simulink model "Control_v2"  (R2019b)
settings: Solver=FixedStepAuto  StartTime=0.0  StopTime=10  FixedStep=str2num(Step_size)  RelTol=1e-3
model workspace: external: MATLAB File H:\4-project\matlab\github\Sim-v2\bicopter_sim\Bicopter_DataFile14.m (data not in the file)
values from neighbouring files (symbols this model uses):
  b = [5,1,5,4]    [init_ADRC_val.m]    (also in init_Non_Linear_ADRC_val.m = 0.5*[1,    1, 6,  6]')
  b_sep = gains(5:8)    [get_ADRC_parameters.m]    (also in get_adrc_sep.m = [  2   7    6   7]; get_adrc_sep_kalman.m = [  2   2    6   7])
  C = [eye(4),zeros(4,8)]    [init_ADRC_val.m]
  C_air = 0.0025    [Sim_Script.m]
  d_f_phi = 100    [Sim_Script.m]
  d_f_psi = 25    [Sim_Script.m]
  d_f_theta = 10    [Sim_Script.m]
  d_f_z = 100    [Sim_Script.m]
  eps_sep = 0.7*[1 1 1 1]    [get_ADRC_parameters.m]    (also in get_adrc_sep.m = [0.7 0.3 0.3 0.35]; get_adrc_sep_kalman.m = [0.7 0.7 0.3 0.35])
  epsi = 1.5    [init_Non_Linear_ADRC_val.m]
  euler_source = 1    [Sim_Script.m]
  freq_cut_angvel_phi = 75    [Sim_Script.m]
  freq_cut_angvel_psi = 75    [Sim_Script.m]
  freq_cut_angvel_theta = 50    [Sim_Script.m]
  g = 9.81    [Sim_Script.m]
  K = place(A1,B1,w00(1:8))    [init_ADRC_val.m]
  L = place(A',C',8*w00)'    [init_ADRC_val.m]
  method = STSC_controller    (= 2)    [Sim_Script.m]
  method_angle_plane_sw = plane_sw    (= 2)    [Sim_Script.m]
  mult_obs = 10    [init_Non_Linear_ADRC_val.m]
  Noise_gain = 1    [Sim_Script.m]
  PID_VAL_SEP = init_pid_val_sep()    [Sim_Script.m]
  polarity = [-1;1;1;1]    [Sim_Script.m]
  r = [10,5,10,10]    [init_Non_Linear_ADRC_val.m]
  S_phi = 0.001    [Sim_Script.m]
  S_psi = S_phi    (= 0.001)    [Sim_Script.m]
  S_theta = S_phi    (= 0.001)    [Sim_Script.m]
  State_step = [Z_step;Phi_step;Theta_step;Psi_step]    [req_response.m]
  Step_size = step_size    [Sim_Script.m]
  STSC_VAL = init_STSC_val()    [Sim_Script.m]
  time_delay = 1e-6    (= 1e-06)    [Sim_Script.m]
  V_phi = 0.01    [Sim_Script.m]
  V_psi = 0.01    [Sim_Script.m]
  V_theta = 0.01    [Sim_Script.m]
  wc_sep = gains(1:4)    [get_ADRC_parameters.m]    (also in get_adrc_sep.m = [ 5.54   9   6    3]; get_adrc_sep_kalman.m = [ 5.54   9   6    3])
  wo_sep = ga*wc_sep    [get_ADRC_parameters.m]    (also in get_adrc_sep.m; get_adrc_sep_kalman.m)
undefined symbols (not defined in the file or in its folder): Continuous, magnitude, NLADRC_VAL, sigbuilder_block, smiData, Time, X, Y, Z
libraries: sm_lib x141, nesl_utility x20, simulink x19, fuzblock x3, sharedtransform x1, ctrlSharedLib x1
(part 6 of 7)

== system Control_v2/System/Controller/fuzzy logic/inner_loop1 ==
  note: Scope_P
  err : Inport
  y_dot : Inport  Port=2
  Derivative : Derivative
  Gain : Gain  Gain=PID_VAL_SEP(parm_id,3)
  Gain1 : Gain  Gain=PID_VAL_SEP(parm_id,3)
  Gain2 : Gain  Gain=PID_VAL_SEP(parm_id,2)
  I : simulink/Continuous/PID Controller  Controller=PID  Form=Parallel  TimeDomain=Continuous-time  SampleTime=-1  IntegratorMethod=Forward Euler  FilterMethod=Forward Euler  ControllerParametersSource=internal  P=0  I=PID_VAL_SEP(parm_id,2)  D=0  UseFilter=on  N=0  TunerSelectOption=Transfer Function Based (PID Tuner App)  InitialConditionSource=internal  InitialConditionForIntegrator=0  InitialConditionForFilter=0  DifferentiatorICPrevScaledInput=0  ExternalReset=none  TrackingMode=off  Kt=1  LimitOutput=off  UpperSaturationLimit=inf  LowerSaturationLimit=-inf  LinearizeAsGain=on  AntiWindupMode=none  Kb=1  POutMin=[]  POutMax=[]  IOutMin=[]  IOutMax=[]  DOutMin=[]  DOutMax=[]  NOutMin=[]  NOutMax=[]  SumOutMin=[]  SumOutMax=[]  SaturationOutMin=[]  SaturationOutMax=[]  PParamMin=[]  PParamMax=[]  IParamMin=[]  IParamMax=[]  DParamMin=[]  DParamMax=[]  NParamMin=[]  NParamMax=[]  KbParamMin=[]  KbParamMax=[]  KtParamMin=[]  KtParamMax=[]  KbOutMin=[]  KbOutMax=[]  KtOutMin=[]  KtOutMax=[]  IntegratorOutMin=[]  IntegratorOutMax=[]  FilterOutMin=[]  FilterOutMax=[]  SumI1OutMin=[]  SumI1OutMax=[]  SumI2OutMin=[]  SumI2OutMax=[]  SumI3OutMin=[]  SumI3OutMax=[]  SumI4OutMin=[]  SumI4OutMax=[]  SumDOutMin=[]  SumDOutMax=[]  DifferentiatorOutMin=[]  DifferentiatorOutMax=[]  FilterDiffOutCoefMin=[]  FilterDiffOutCoefMax=[]  ReciprocalOutMin=[]  ReciprocalOutMax=[]  SumDenOutMin=[]  SumDenOutMax=[]  SumNumOutMin=[]  SumNumOutMax=[]  DivideOutMin=[]  DivideOutMax=[]  IntegratorContinuousStateAttributes=''  IntegratorStateMustResolveToSignalObject=off  IntegratorRTWStateStorageClass=Auto  FilterContinuousStateAttributes=''  FilterStateMustResolveToSignalObject=off  FilterRTWStateStorageClass=Auto  ParallelPVariant=InternalParameters  IdealPVariant=Disabled  IVariant=InternalParameters  DVariant=InternalParameters  IntegratorVariant=Continuous  SatVariant=Disabled  AWVariant=Passthrough  PCopyVariant=Disabled  TRVariant=Disabled  FdbkBlocksVariant=Forward  IdealPFdbkVariant=Disabled  SatFdbkVariant=Disabled  DerivativeFilterVariant=ContFilter  NVariant=InternalParameters  NCopyVariant=Disabled  FilterICVariant=InternalICsFilter  IntegratorICVariant=InternalICs  ExternalResetVariant=Disabled  TRSumVariant=Passthrough  SumFdbkVariant=Disabled  SumVariant=Sum_PID
  Integrator Limited : Integrator  LimitOutput=on  UpperSaturationLimit=5  LowerSaturationLimit=-5
  P : simulink/Continuous/PID Controller  Controller=PID  Form=Parallel  TimeDomain=Continuous-time  SampleTime=-1  IntegratorMethod=Forward Euler  FilterMethod=Forward Euler  ControllerParametersSource=internal  P=PID_VAL_SEP(parm_id,1)  I=0  D=0  UseFilter=on  N=0  TunerSelectOption=Transfer Function Based (PID Tuner App)  InitialConditionSource=internal  InitialConditionForIntegrator=0  InitialConditionForFilter=0  DifferentiatorICPrevScaledInput=0  ExternalReset=none  TrackingMode=off  Kt=1  LimitOutput=off  UpperSaturationLimit=inf  LowerSaturationLimit=-inf  LinearizeAsGain=on  AntiWindupMode=none  Kb=1  POutMin=[]  POutMax=[]  IOutMin=[]  IOutMax=[]  DOutMin=[]  DOutMax=[]  NOutMin=[]  NOutMax=[]  SumOutMin=[]  SumOutMax=[]  SaturationOutMin=[]  SaturationOutMax=[]  PParamMin=[]  PParamMax=[]  IParamMin=[]  IParamMax=[]  DParamMin=[]  DParamMax=[]  NParamMin=[]  NParamMax=[]  KbParamMin=[]  KbParamMax=[]  KtParamMin=[]  KtParamMax=[]  KbOutMin=[]  KbOutMax=[]  KtOutMin=[]  KtOutMax=[]  IntegratorOutMin=[]  IntegratorOutMax=[]  FilterOutMin=[]  FilterOutMax=[]  SumI1OutMin=[]  SumI1OutMax=[]  SumI2OutMin=[]  SumI2OutMax=[]  SumI3OutMin=[]  SumI3OutMax=[]  SumI4OutMin=[]  SumI4OutMax=[]  SumDOutMin=[]  SumDOutMax=[]  DifferentiatorOutMin=[]  DifferentiatorOutMax=[]  FilterDiffOutCoefMin=[]  FilterDiffOutCoefMax=[]  ReciprocalOutMin=[]  ReciprocalOutMax=[]  SumDenOutMin=[]  SumDenOutMax=[]  SumNumOutMin=[]  SumNumOutMax=[]  DivideOutMin=[]  DivideOutMax=[]  IntegratorContinuousStateAttributes=''  IntegratorStateMustResolveToSignalObject=off  IntegratorRTWStateStorageClass=Auto  FilterContinuousStateAttributes=''  FilterStateMustResolveToSignalObject=off  FilterRTWStateStorageClass=Auto  ParallelPVariant=InternalParameters  IdealPVariant=Disabled  IVariant=InternalParameters  DVariant=InternalParameters  IntegratorVariant=Continuous  SatVariant=Disabled  AWVariant=Passthrough  PCopyVariant=Disabled  TRVariant=Disabled  FdbkBlocksVariant=Forward  IdealPFdbkVariant=Disabled  SatFdbkVariant=Disabled  DerivativeFilterVariant=ContFilter  NVariant=InternalParameters  NCopyVariant=Disabled  FilterICVariant=InternalICsFilter  IntegratorICVariant=InternalICs  ExternalResetVariant=Disabled  TRSumVariant=Passthrough  SumFdbkVariant=Disabled  SumVariant=Sum_PID
  Scope : Scope  NumInputPorts=2
  Scope1 : Scope  NumInputPorts=2
  Scope_D : Scope  NumInputPorts=2
  Scope_D1 : Scope  NumInputPorts=2
  Scope_I : Scope  NumInputPorts=2
  Sum : Sum  Inputs=|+++-
  Transfer Fcn : TransferFcn  Numerator=[2*pi*f]  Denominator=[1 2*pi*f]
  Transfer Fcn1 : TransferFcn  Numerator=[2*pi*f]  Denominator=[1 2*pi*f]
  phiCmd : Scope  NumInputPorts=2
  cmd : Outport
  wires:
  Sum/1 -> phiCmd/2, cmd/1  "after"
  y_dot/1 -> Gain/1, Scope_D/1
  err/1 -> Gain2/1, Gain1/1, I/1, Scope_I/2, P/1, Scope/1, phiCmd/1  "err"
  P/1 -> Sum/1, Scope/2
  I/1 -> Scope1/2, Scope_I/1
  Gain1/1 -> Derivative/1  "before"
  Derivative/1 -> Transfer Fcn/1
  Gain/1 -> Sum/4, Transfer Fcn1/1  "before"
  Gain2/1 -> Integrator Limited/1
  Integrator Limited/1 -> Scope1/1, Sum/3

== system Control_v2/System/Controller/fuzzy logic/inner_loop2 ==
  note: Scope_P
  err : Inport
  y_dot : Inport  Port=2
  Derivative : Derivative
  Gain : Gain  Gain=PID_VAL_SEP(parm_id,3)
  Gain1 : Gain  Gain=PID_VAL_SEP(parm_id,3)
  I : simulink/Continuous/PID Controller  Controller=PID  Form=Parallel  TimeDomain=Continuous-time  SampleTime=-1  IntegratorMethod=Forward Euler  FilterMethod=Forward Euler  ControllerParametersSource=internal  P=0  I=PID_VAL_SEP(parm_id,2)  D=0  UseFilter=on  N=0  TunerSelectOption=Transfer Function Based (PID Tuner App)  InitialConditionSource=internal  InitialConditionForIntegrator=0  InitialConditionForFilter=0  DifferentiatorICPrevScaledInput=0  ExternalReset=none  TrackingMode=off  Kt=1  LimitOutput=off  UpperSaturationLimit=inf  LowerSaturationLimit=-inf  LinearizeAsGain=on  AntiWindupMode=none  Kb=1  POutMin=[]  POutMax=[]  IOutMin=[]  IOutMax=[]  DOutMin=[]  DOutMax=[]  NOutMin=[]  NOutMax=[]  SumOutMin=[]  SumOutMax=[]  SaturationOutMin=[]  SaturationOutMax=[]  PParamMin=[]  PParamMax=[]  IParamMin=[]  IParamMax=[]  DParamMin=[]  DParamMax=[]  NParamMin=[]  NParamMax=[]  KbParamMin=[]  KbParamMax=[]  KtParamMin=[]  KtParamMax=[]  KbOutMin=[]  KbOutMax=[]  KtOutMin=[]  KtOutMax=[]  IntegratorOutMin=[]  IntegratorOutMax=[]  FilterOutMin=[]  FilterOutMax=[]  SumI1OutMin=[]  SumI1OutMax=[]  SumI2OutMin=[]  SumI2OutMax=[]  SumI3OutMin=[]  SumI3OutMax=[]  SumI4OutMin=[]  SumI4OutMax=[]  SumDOutMin=[]  SumDOutMax=[]  DifferentiatorOutMin=[]  DifferentiatorOutMax=[]  FilterDiffOutCoefMin=[]  FilterDiffOutCoefMax=[]  ReciprocalOutMin=[]  ReciprocalOutMax=[]  SumDenOutMin=[]  SumDenOutMax=[]  SumNumOutMin=[]  SumNumOutMax=[]  DivideOutMin=[]  DivideOutMax=[]  IntegratorContinuousStateAttributes=''  IntegratorStateMustResolveToSignalObject=off  IntegratorRTWStateStorageClass=Auto  FilterContinuousStateAttributes=''  FilterStateMustResolveToSignalObject=off  FilterRTWStateStorageClass=Auto  ParallelPVariant=InternalParameters  IdealPVariant=Disabled  IVariant=InternalParameters  DVariant=InternalParameters  IntegratorVariant=Continuous  SatVariant=Disabled  AWVariant=Passthrough  PCopyVariant=Disabled  TRVariant=Disabled  FdbkBlocksVariant=Forward  IdealPFdbkVariant=Disabled  SatFdbkVariant=Disabled  DerivativeFilterVariant=ContFilter  NVariant=InternalParameters  NCopyVariant=Disabled  FilterICVariant=InternalICsFilter  IntegratorICVariant=InternalICs  ExternalResetVariant=Disabled  TRSumVariant=Passthrough  SumFdbkVariant=Disabled  SumVariant=Sum_PID
  P : simulink/Continuous/PID Controller  Controller=PID  Form=Parallel  TimeDomain=Continuous-time  SampleTime=-1  IntegratorMethod=Forward Euler  FilterMethod=Forward Euler  ControllerParametersSource=internal  P=PID_VAL_SEP(parm_id,1)  I=0  D=0  UseFilter=on  N=0  TunerSelectOption=Transfer Function Based (PID Tuner App)  InitialConditionSource=internal  InitialConditionForIntegrator=0  InitialConditionForFilter=0  DifferentiatorICPrevScaledInput=0  ExternalReset=none  TrackingMode=off  Kt=1  LimitOutput=off  UpperSaturationLimit=inf  LowerSaturationLimit=-inf  LinearizeAsGain=on  AntiWindupMode=none  Kb=1  POutMin=[]  POutMax=[]  IOutMin=[]  IOutMax=[]  DOutMin=[]  DOutMax=[]  NOutMin=[]  NOutMax=[]  SumOutMin=[]  SumOutMax=[]  SaturationOutMin=[]  SaturationOutMax=[]  PParamMin=[]  PParamMax=[]  IParamMin=[]  IParamMax=[]  DParamMin=[]  DParamMax=[]  NParamMin=[]  NParamMax=[]  KbParamMin=[]  KbParamMax=[]  KtParamMin=[]  KtParamMax=[]  KbOutMin=[]  KbOutMax=[]  KtOutMin=[]  KtOutMax=[]  IntegratorOutMin=[]  IntegratorOutMax=[]  FilterOutMin=[]  FilterOutMax=[]  SumI1OutMin=[]  SumI1OutMax=[]  SumI2OutMin=[]  SumI2OutMax=[]  SumI3OutMin=[]  SumI3OutMax=[]  SumI4OutMin=[]  SumI4OutMax=[]  SumDOutMin=[]  SumDOutMax=[]  DifferentiatorOutMin=[]  DifferentiatorOutMax=[]  FilterDiffOutCoefMin=[]  FilterDiffOutCoefMax=[]  ReciprocalOutMin=[]  ReciprocalOutMax=[]  SumDenOutMin=[]  SumDenOutMax=[]  SumNumOutMin=[]  SumNumOutMax=[]  DivideOutMin=[]  DivideOutMax=[]  IntegratorContinuousStateAttributes=''  IntegratorStateMustResolveToSignalObject=off  IntegratorRTWStateStorageClass=Auto  FilterContinuousStateAttributes=''  FilterStateMustResolveToSignalObject=off  FilterRTWStateStorageClass=Auto  ParallelPVariant=InternalParameters  IdealPVariant=Disabled  IVariant=InternalParameters  DVariant=InternalParameters  IntegratorVariant=Continuous  SatVariant=Disabled  AWVariant=Passthrough  PCopyVariant=Disabled  TRVariant=Disabled  FdbkBlocksVariant=Forward  IdealPFdbkVariant=Disabled  SatFdbkVariant=Disabled  DerivativeFilterVariant=ContFilter  NVariant=InternalParameters  NCopyVariant=Disabled  FilterICVariant=InternalICsFilter  IntegratorICVariant=InternalICs  ExternalResetVariant=Disabled  TRSumVariant=Passthrough  SumFdbkVariant=Disabled  SumVariant=Sum_PID
  Scope : Scope  NumInputPorts=2
  Scope_D : Scope  NumInputPorts=2
  Scope_D1 : Scope  NumInputPorts=2
  Scope_I : Scope  NumInputPorts=2
  Sum : Sum  Inputs=|+++-
  Transfer Fcn : TransferFcn  Numerator=[2*pi*f]  Denominator=[1 2*pi*f]
  Transfer Fcn1 : TransferFcn  Numerator=[2*pi*f]  Denominator=[1 2*pi*f]
  phiCmd : Scope  NumInputPorts=2
  cmd : Outport
  wires:
  Gain/1 -> Transfer Fcn1/1  "before"
  I/1 -> Scope_I/1, Sum/2
  P/1 -> Scope/2, Sum/1
  err/1 -> phiCmd/1, Gain1/1, Scope/1, P/1, Scope_I/2, I/1  "err"
  y_dot/1 -> Gain/1
  Sum/1 -> cmd/1, phiCmd/2  "after"
  Derivative/1 -> Scope_D/2, Transfer Fcn/1
  Gain1/1 -> Derivative/1  "before"
  Transfer Fcn/1 -> Scope_D/1  "after"
  Transfer Fcn1/1 -> Scope_D1/2, Sum/4  "after"

== system Control_v2/System/Controller/fuzzy logic/inner_loop4 ==
  note: Scope_P
  err : Inport
  y_dot : Inport  Port=2
  Derivative : Derivative
  Gain : Gain  Gain=PID_VAL_SEP(parm_id,3)
  Gain1 : Gain  Gain=PID_VAL_SEP(parm_id,3)
  I : simulink/Continuous/PID Controller  Controller=PID  Form=Parallel  TimeDomain=Continuous-time  SampleTime=-1  IntegratorMethod=Forward Euler  FilterMethod=Forward Euler  ControllerParametersSource=internal  P=0  I=PID_VAL_SEP(parm_id,2)  D=0  UseFilter=on  N=0  TunerSelectOption=Transfer Function Based (PID Tuner App)  InitialConditionSource=internal  InitialConditionForIntegrator=0  InitialConditionForFilter=0  DifferentiatorICPrevScaledInput=0  ExternalReset=none  TrackingMode=off  Kt=1  LimitOutput=off  UpperSaturationLimit=inf  LowerSaturationLimit=-inf  LinearizeAsGain=on  AntiWindupMode=none  Kb=1  POutMin=[]  POutMax=[]  IOutMin=[]  IOutMax=[]  DOutMin=[]  DOutMax=[]  NOutMin=[]  NOutMax=[]  SumOutMin=[]  SumOutMax=[]  SaturationOutMin=[]  SaturationOutMax=[]  PParamMin=[]  PParamMax=[]  IParamMin=[]  IParamMax=[]  DParamMin=[]  DParamMax=[]  NParamMin=[]  NParamMax=[]  KbParamMin=[]  KbParamMax=[]  KtParamMin=[]  KtParamMax=[]  KbOutMin=[]  KbOutMax=[]  KtOutMin=[]  KtOutMax=[]  IntegratorOutMin=[]  IntegratorOutMax=[]  FilterOutMin=[]  FilterOutMax=[]  SumI1OutMin=[]  SumI1OutMax=[]  SumI2OutMin=[]  SumI2OutMax=[]  SumI3OutMin=[]  SumI3OutMax=[]  SumI4OutMin=[]  SumI4OutMax=[]  SumDOutMin=[]  SumDOutMax=[]  DifferentiatorOutMin=[]  DifferentiatorOutMax=[]  FilterDiffOutCoefMin=[]  FilterDiffOutCoefMax=[]  ReciprocalOutMin=[]  ReciprocalOutMax=[]  SumDenOutMin=[]  SumDenOutMax=[]  SumNumOutMin=[]  SumNumOutMax=[]  DivideOutMin=[]  DivideOutMax=[]  IntegratorContinuousStateAttributes=''  IntegratorStateMustResolveToSignalObject=off  IntegratorRTWStateStorageClass=Auto  FilterContinuousStateAttributes=''  FilterStateMustResolveToSignalObject=off  FilterRTWStateStorageClass=Auto  ParallelPVariant=InternalParameters  IdealPVariant=Disabled  IVariant=InternalParameters  DVariant=InternalParameters  IntegratorVariant=Continuous  SatVariant=Disabled  AWVariant=Passthrough  PCopyVariant=Disabled  TRVariant=Disabled  FdbkBlocksVariant=Forward  IdealPFdbkVariant=Disabled  SatFdbkVariant=Disabled  DerivativeFilterVariant=ContFilter  NVariant=InternalParameters  NCopyVariant=Disabled  FilterICVariant=InternalICsFilter  IntegratorICVariant=InternalICs  ExternalResetVariant=Disabled  TRSumVariant=Passthrough  SumFdbkVariant=Disabled  SumVariant=Sum_PID
  P : simulink/Continuous/PID Controller  Controller=PID  Form=Parallel  TimeDomain=Continuous-time  SampleTime=-1  IntegratorMethod=Forward Euler  FilterMethod=Forward Euler  ControllerParametersSource=internal  P=PID_VAL_SEP(parm_id,1)  I=0  D=0  UseFilter=on  N=0  TunerSelectOption=Transfer Function Based (PID Tuner App)  InitialConditionSource=internal  InitialConditionForIntegrator=0  InitialConditionForFilter=0  DifferentiatorICPrevScaledInput=0  ExternalReset=none  TrackingMode=off  Kt=1  LimitOutput=off  UpperSaturationLimit=inf  LowerSaturationLimit=-inf  LinearizeAsGain=on  AntiWindupMode=none  Kb=1  POutMin=[]  POutMax=[]  IOutMin=[]  IOutMax=[]  DOutMin=[]  DOutMax=[]  NOutMin=[]  NOutMax=[]  SumOutMin=[]  SumOutMax=[]  SaturationOutMin=[]  SaturationOutMax=[]  PParamMin=[]  PParamMax=[]  IParamMin=[]  IParamMax=[]  DParamMin=[]  DParamMax=[]  NParamMin=[]  NParamMax=[]  KbParamMin=[]  KbParamMax=[]  KtParamMin=[]  KtParamMax=[]  KbOutMin=[]  KbOutMax=[]  KtOutMin=[]  KtOutMax=[]  IntegratorOutMin=[]  IntegratorOutMax=[]  FilterOutMin=[]  FilterOutMax=[]  SumI1OutMin=[]  SumI1OutMax=[]  SumI2OutMin=[]  SumI2OutMax=[]  SumI3OutMin=[]  SumI3OutMax=[]  SumI4OutMin=[]  SumI4OutMax=[]  SumDOutMin=[]  SumDOutMax=[]  DifferentiatorOutMin=[]  DifferentiatorOutMax=[]  FilterDiffOutCoefMin=[]  FilterDiffOutCoefMax=[]  ReciprocalOutMin=[]  ReciprocalOutMax=[]  SumDenOutMin=[]  SumDenOutMax=[]  SumNumOutMin=[]  SumNumOutMax=[]  DivideOutMin=[]  DivideOutMax=[]  IntegratorContinuousStateAttributes=''  IntegratorStateMustResolveToSignalObject=off  IntegratorRTWStateStorageClass=Auto  FilterContinuousStateAttributes=''  FilterStateMustResolveToSignalObject=off  FilterRTWStateStorageClass=Auto  ParallelPVariant=InternalParameters  IdealPVariant=Disabled  IVariant=InternalParameters  DVariant=InternalParameters  IntegratorVariant=Continuous  SatVariant=Disabled  AWVariant=Passthrough  PCopyVariant=Disabled  TRVariant=Disabled  FdbkBlocksVariant=Forward  IdealPFdbkVariant=Disabled  SatFdbkVariant=Disabled  DerivativeFilterVariant=ContFilter  NVariant=InternalParameters  NCopyVariant=Disabled  FilterICVariant=InternalICsFilter  IntegratorICVariant=InternalICs  ExternalResetVariant=Disabled  TRSumVariant=Passthrough  SumFdbkVariant=Disabled  SumVariant=Sum_PID
  Scope : Scope  NumInputPorts=2
  Scope_D : Scope  NumInputPorts=2
  Scope_D1 : Scope  NumInputPorts=2
  Scope_I : Scope  NumInputPorts=2
  Sum : Sum  Inputs=|+++-
  Transfer Fcn : TransferFcn  Numerator=[2*pi*f]  Denominator=[1 2*pi*f]
  Transfer Fcn1 : TransferFcn  Numerator=[2*pi*f]  Denominator=[1 2*pi*f]
  phiCmd : Scope  NumInputPorts=2
  cmd : Outport
  wires:
  Gain/1 -> Sum/4, Transfer Fcn1/1  "before"
  I/1 -> Scope_I/1, Sum/2
  P/1 -> Scope/2, Sum/1
  err/1 -> Gain1/1, Scope/1, P/1, Scope_I/2, I/1, phiCmd/1  "err"
  y_dot/1 -> Gain/1
  Sum/1 -> cmd/1, phiCmd/2  "after"
  Derivative/1 -> Scope_D/2, Transfer Fcn/1
  Gain1/1 -> Derivative/1  "before"
  Transfer Fcn/1 -> Scope_D/1  "after"
  Transfer Fcn1/1 -> Scope_D1/2  "after"

== system Control_v2/System/Controller/fuzzy logic/inner_loop7 ==
  note: Scope_P
  err : Inport
  y_dot : Inport  Port=2
  Derivative : Derivative
  Gain : Gain  Gain=PID_VAL_SEP(parm_id,3)
  Gain1 : Gain  Gain=PID_VAL_SEP(parm_id,3)
  Gain2 : Gain  Gain=PID_VAL_SEP(parm_id,2)
  I : simulink/Continuous/PID Controller  Controller=PID  Form=Parallel  TimeDomain=Continuous-time  SampleTime=-1  IntegratorMethod=Forward Euler  FilterMethod=Forward Euler  ControllerParametersSource=internal  P=0  I=PID_VAL_SEP(parm_id,2)  D=0  UseFilter=on  N=100  TunerSelectOption=Transfer Function Based (PID Tuner App)  InitialConditionSource=internal  InitialConditionForIntegrator=0  InitialConditionForFilter=0  DifferentiatorICPrevScaledInput=0  ExternalReset=none  TrackingMode=off  Kt=1  LimitOutput=off  UpperSaturationLimit=inf  LowerSaturationLimit=-inf  LinearizeAsGain=on  AntiWindupMode=none  Kb=1  POutMin=[]  POutMax=[]  IOutMin=[]  IOutMax=[]  DOutMin=[]  DOutMax=[]  NOutMin=[]  NOutMax=[]  SumOutMin=[]  SumOutMax=[]  SaturationOutMin=[]  SaturationOutMax=[]  PParamMin=[]  PParamMax=[]  IParamMin=[]  IParamMax=[]  DParamMin=[]  DParamMax=[]  NParamMin=[]  NParamMax=[]  KbParamMin=[]  KbParamMax=[]  KtParamMin=[]  KtParamMax=[]  KbOutMin=[]  KbOutMax=[]  KtOutMin=[]  KtOutMax=[]  IntegratorOutMin=[]  IntegratorOutMax=[]  FilterOutMin=[]  FilterOutMax=[]  SumI1OutMin=[]  SumI1OutMax=[]  SumI2OutMin=[]  SumI2OutMax=[]  SumI3OutMin=[]  SumI3OutMax=[]  SumI4OutMin=[]  SumI4OutMax=[]  SumDOutMin=[]  SumDOutMax=[]  DifferentiatorOutMin=[]  DifferentiatorOutMax=[]  FilterDiffOutCoefMin=[]  FilterDiffOutCoefMax=[]  ReciprocalOutMin=[]  ReciprocalOutMax=[]  SumDenOutMin=[]  SumDenOutMax=[]  SumNumOutMin=[]  SumNumOutMax=[]  DivideOutMin=[]  DivideOutMax=[]  IntegratorContinuousStateAttributes=''  IntegratorStateMustResolveToSignalObject=off  IntegratorRTWStateStorageClass=Auto  FilterContinuousStateAttributes=''  FilterStateMustResolveToSignalObject=off  FilterRTWStateStorageClass=Auto  ParallelPVariant=InternalParameters  IdealPVariant=Disabled  IVariant=InternalParameters  DVariant=InternalParameters  IntegratorVariant=Continuous  SatVariant=Disabled  AWVariant=Passthrough  PCopyVariant=Disabled  TRVariant=Disabled  FdbkBlocksVariant=Forward  IdealPFdbkVariant=Disabled  SatFdbkVariant=Disabled  DerivativeFilterVariant=ContFilter  NVariant=InternalParameters  NCopyVariant=Disabled  FilterICVariant=InternalICsFilter  IntegratorICVariant=InternalICs  ExternalResetVariant=Disabled  TRSumVariant=Passthrough  SumFdbkVariant=Disabled  SumVariant=Sum_PID
  Integrator Limited : Integrator  LimitOutput=on  UpperSaturationLimit=0.5  LowerSaturationLimit=-0.5
  P : simulink/Continuous/PID Controller  Controller=PID  Form=Parallel  TimeDomain=Continuous-time  SampleTime=-1  IntegratorMethod=Forward Euler  FilterMethod=Forward Euler  ControllerParametersSource=internal  P=PID_VAL_SEP(parm_id,1)  I=0  D=0  UseFilter=on  N=100  TunerSelectOption=Transfer Function Based (PID Tuner App)  InitialConditionSource=internal  InitialConditionForIntegrator=0  InitialConditionForFilter=0  DifferentiatorICPrevScaledInput=0  ExternalReset=none  TrackingMode=off  Kt=1  LimitOutput=off  UpperSaturationLimit=inf  LowerSaturationLimit=-inf  LinearizeAsGain=on  AntiWindupMode=none  Kb=1  POutMin=[]  POutMax=[]  IOutMin=[]  IOutMax=[]  DOutMin=[]  DOutMax=[]  NOutMin=[]  NOutMax=[]  SumOutMin=[]  SumOutMax=[]  SaturationOutMin=[]  SaturationOutMax=[]  PParamMin=[]  PParamMax=[]  IParamMin=[]  IParamMax=[]  DParamMin=[]  DParamMax=[]  NParamMin=[]  NParamMax=[]  KbParamMin=[]  KbParamMax=[]  KtParamMin=[]  KtParamMax=[]  KbOutMin=[]  KbOutMax=[]  KtOutMin=[]  KtOutMax=[]  IntegratorOutMin=[]  IntegratorOutMax=[]  FilterOutMin=[]  FilterOutMax=[]  SumI1OutMin=[]  SumI1OutMax=[]  SumI2OutMin=[]  SumI2OutMax=[]  SumI3OutMin=[]  SumI3OutMax=[]  SumI4OutMin=[]  SumI4OutMax=[]  SumDOutMin=[]  SumDOutMax=[]  DifferentiatorOutMin=[]  DifferentiatorOutMax=[]  FilterDiffOutCoefMin=[]  FilterDiffOutCoefMax=[]  ReciprocalOutMin=[]  ReciprocalOutMax=[]  SumDenOutMin=[]  SumDenOutMax=[]  SumNumOutMin=[]  SumNumOutMax=[]  DivideOutMin=[]  DivideOutMax=[]  IntegratorContinuousStateAttributes=''  IntegratorStateMustResolveToSignalObject=off  IntegratorRTWStateStorageClass=Auto  FilterContinuousStateAttributes=''  FilterStateMustResolveToSignalObject=off  FilterRTWStateStorageClass=Auto  ParallelPVariant=InternalParameters  IdealPVariant=Disabled  IVariant=InternalParameters  DVariant=InternalParameters  IntegratorVariant=Continuous  SatVariant=Disabled  AWVariant=Passthrough  PCopyVariant=Disabled  TRVariant=Disabled  FdbkBlocksVariant=Forward  IdealPFdbkVariant=Disabled  SatFdbkVariant=Disabled  DerivativeFilterVariant=ContFilter  NVariant=InternalParameters  NCopyVariant=Disabled  FilterICVariant=InternalICsFilter  IntegratorICVariant=InternalICs  ExternalResetVariant=Disabled  TRSumVariant=Passthrough  SumFdbkVariant=Disabled  SumVariant=Sum_PID
  Scope : Scope  NumInputPorts=2
  Scope1 : Scope  NumInputPorts=2
  Scope2 : Scope  NumInputPorts=4
  Scope_D : Scope  NumInputPorts=2
  Scope_D1 : Scope  NumInputPorts=2
  Scope_I : Scope  NumInputPorts=2
  Sum : Sum  Inputs=|+++-
  Sum1 : Sum  Inputs=|+-
  Transfer Fcn : TransferFcn  Numerator=[2*pi*f]  Denominator=[1 2*pi*f]
  Transfer Fcn1 : TransferFcn  Numerator=[2*pi*f]  Denominator=[1 2*pi*f]
  cmd : Outport
  wires:
  I/1 -> Scope_I/1
  P/1 -> Scope/2, Scope2/1, Sum/1
  err/1 -> Gain2/1, Gain1/1, Sum1/1
  Sum1/1 -> Scope1/1, Scope/1, P/1, Scope_I/2, I/1
  Gain/1 -> Sum/4, Scope2/3, Scope_D1/2, Transfer Fcn1/1  "before"
  Sum/1 -> Scope2/4, Scope1/2, cmd/1  "after"
  y_dot/1 -> Gain/1, Scope_D/1  "after"
  Gain1/1 -> Derivative/1  "before"
  Derivative/1 -> Transfer Fcn/1
  Gain2/1 -> Integrator Limited/1
  Integrator Limited/1 -> Scope2/2, Sum/3

== system Control_v2/System/Controller/super_twisting_controller1/STSC_PSI ==
  error : Inport
  error_dot : Inport  Port=2
  Abs : Abs
  Add : Sum
  Derivative : Derivative  Commented=on
  Gain : Gain  Gain=STSC_VAL(parm_id,2)
  Gain1 : Gain  Gain=1/STSC_VAL(parm_id,1)
  Gain2 : Gain  Gain=STSC_VAL(parm_id,3)
  Integrator : Integrator
  Product : Product
  Saturation : Saturate  UpperLimit=0.3  LowerLimit=-0.3
  Sign : Signum
  Sqrt : Sqrt  SaturateOnIntegerOverflow=on
  Sum : Sum  Inputs=|++-
  Transfer Fcn : TransferFcn  Commented=on  Numerator=[2*pi*f]  Denominator=[1 2*pi*f]
  Transfer Fcn1 : TransferFcn  Numerator=[2*pi*f]  Denominator=[1 2*pi*f]
  Transfer Fcn2 : TransferFcn  Numerator=[2*pi*f]  Denominator=[1 2*pi*f]
  cmd : Outport
  wires:
  Gain/1 -> Add/1
  Gain2/1 -> Add/2
  Abs/1 -> Sqrt/1
  Product/1 -> Gain/1
  Sqrt/1 -> Product/1
  Integrator/1 -> Gain2/1
  Sign/1 -> Integrator/1, Product/2
  Sum/1 -> Sign/1, Abs/1
  Derivative/1 -> Transfer Fcn/1
  Gain1/1 -> Transfer Fcn2/1
  error/1 -> Derivative/1, Saturation/1
  Saturation/1 -> Sum/1
  error_dot/1 -> Gain1/1
  Add/1 -> Transfer Fcn1/1
  Transfer Fcn1/1 -> cmd/1
  Transfer Fcn2/1 -> Sum/3

== system Control_v2/System/Controller/super_twisting_controller1/STSC_Phi ==
  error : Inport
  error_dot : Inport  Port=2
  Abs : Abs
  Add : Sum
  Derivative : Derivative  Commented=on
  Gain : Gain  Gain=STSC_VAL(parm_id,2)
  Gain1 : Gain  Gain=1/STSC_VAL(parm_id,1)
  Gain2 : Gain  Gain=STSC_VAL(parm_id,3)
  Gain3 : Gain  Gain=PID_VAL_SEP(parm_id,3)
  Integrator : Integrator
  Product : Product
  Scope : Scope  NumInputPorts=4
  Sign : Signum
  Sqrt : Sqrt  SaturateOnIntegerOverflow=on
  Sum : Sum  Inputs=|++-
  Transfer Fcn : TransferFcn  Commented=on  Numerator=[2*pi*f]  Denominator=[1 2*pi*f]
  Transfer Fcn1 : TransferFcn  Numerator=[2*pi*f]  Denominator=[1 2*pi*f]
  cmd : Outport
  wires:
  Sum/1 -> Abs/1, Scope/3, Sign/1
  Sign/1 -> Integrator/1, Product/2
  Integrator/1 -> Gain2/1
  error/1 -> Derivative/1, Scope/1, Sum/1
  Sqrt/1 -> Product/1
  Product/1 -> Gain/1
  Abs/1 -> Sqrt/1
  Gain2/1 -> Add/2
  Gain/1 -> Add/1
  Derivative/1 -> Transfer Fcn/1
  error_dot/1 -> Gain1/1
  Gain1/1 -> Scope/2, Sum/3
  Add/1 -> cmd/1

== system Control_v2/System/Controller/super_twisting_controller1/STSC_Phi2 ==
  error : Inport
  error_dot : Inport  Port=2
  Abs : Abs
  Add : Sum
  Derivative : Derivative  Commented=on
  Gain : Gain  Gain=STSC_VAL(parm_id,2)
  Gain1 : Gain  Gain=1/STSC_VAL(parm_id,1)
  Gain2 : Gain  Gain=STSC_VAL(parm_id,3)
  Gain3 : Gain  Gain=10
  Integrator : Integrator
  MATLAB Function : MATLAB Function  TreatAsAtomicUnit=on
  MATLAB Function1 : MATLAB Function  TreatAsAtomicUnit=on
  Product : Product
  Scope : Scope
  Scope1 : Scope  NumInputPorts=4
  Sign : Signum
  Sqrt : Sqrt  SaturateOnIntegerOverflow=on
  Sum : Sum  Inputs=|++-
  Transfer Fcn : TransferFcn  Commented=on  Numerator=[2*pi*f]  Denominator=[1 2*pi*f]
  Transfer Fcn1 : TransferFcn  Numerator=[2*pi*f]  Denominator=[1 2*pi*f]
  Transfer Fcn2 : TransferFcn  Numerator=[2*pi*f]  Denominator=[1 2*pi*f]
  cmd : Outport
  wires:
  Integrator/1 -> Gain2/1
  Sqrt/1 -> Product/1
  Product/1 -> Gain/1
  Abs/1 -> Sqrt/1
  Gain2/1 -> Add/2
  Gain/1 -> Add/1
  Derivative/1 -> Transfer Fcn/1
  Sum/1 -> Scope1/3, Scope/1, Abs/1, MATLAB Function/1(u), Sign/1
  error/1 -> MATLAB Function1/2(error), Derivative/1, Scope1/1, Sum/1
  Add/1 -> Gain3/1, Scope1/4, Transfer Fcn1/1
  MATLAB Function/1(y) -> Integrator/1, Product/2
  Gain1/1 -> Scope1/2, Sum/3
  error_dot/1 -> Transfer Fcn2/1
  Transfer Fcn2/1 -> Gain1/1  "after"
  Transfer Fcn1/1 -> cmd/1  "after"

== system Control_v2/System/Controller/super_twisting_controller1/STSC_Z ==
  error : Inport
  error_dot : Inport  Port=2
  Abs : Abs
  Add : Sum
  Derivative : Derivative  Commented=on
  Gain : Gain  Gain=STSC_VAL(parm_id,2)
  Gain1 : Gain  Gain=1/STSC_VAL(parm_id,1)
  Gain2 : Gain  Gain=STSC_VAL(parm_id,3)
  Integrator : Integrator
  Product : Product
  Saturation : Saturate  UpperLimit=2  LowerLimit=-2
  Sign : Signum
  Sqrt : Sqrt  SaturateOnIntegerOverflow=on
  Sum : Sum  Inputs=|++-
  Transfer Fcn : TransferFcn  Commented=on  Numerator=[2*pi*f]  Denominator=[1 2*pi*f]
  Transfer Fcn1 : TransferFcn  Numerator=[2*pi*f]  Denominator=[1 2*pi*f]
  cmd : Outport
  wires:
  Gain/1 -> Add/1
  Gain2/1 -> Add/2
  Abs/1 -> Sqrt/1
  Product/1 -> Gain/1
  Sqrt/1 -> Product/1
  error/1 -> Derivative/1, Saturation/1
  Integrator/1 -> Gain2/1
  Sign/1 -> Integrator/1, Product/2
  Sum/1 -> Sign/1, Abs/1
  Derivative/1 -> Transfer Fcn/1
  error_dot/1 -> Gain1/1
  Gain1/1 -> Sum/3
  Saturation/1 -> Sum/1
  Add/1 -> cmd/1

== system Control_v2/System/Controller/ADRC_Kalman/Phi_loop/LESO ==
  y : Inport
  u : Inport  Port=2
  Add : Sum  Inputs=+++
  Gain : Gain  Gain=3*wo_sep(ind)
  Gain1 : Gain  Gain=3*(wo_sep(ind))^2
  Gain2 : Gain  Gain=wo_sep(ind)^3
  Integrator : Integrator
  Integrator Limited : Integrator  LimitOutput=on  UpperSaturationLimit=3  LowerSaturationLimit=-3
  Integrator1 : Integrator
  Integrator2 : Integrator
  Scope : Scope
  Sum : Sum  Inputs=|+-
  Sum1 : Sum  Inputs=|++
  Z1 : Outport
  Z2 : Outport  Port=2
  Z3 : Outport  Port=3
  wires:
  Integrator1/1 -> Z2/1, [Z2]
  [Z3] -> Add/1
  y/1 -> Sum/1
  u/1 -> Add/2
  Integrator/1 -> Z1/1, [Z1]
  Sum/1 -> Gain2/1, Gain1/1, Gain/1
  Add/1 -> Integrator1/1
  [Z2] -> Sum1/2
  Sum1/1 -> Integrator/1
  Gain1/1 -> Add/3
  Gain2/1 -> Integrator2/1
  [Z1] -> Sum/2
  Gain/1 -> Sum1/1
  Integrator2/1 -> Scope/1, Z3/1, [Z3]

== system Control_v2/System/Controller/ADRC_Kalman/Z_loop/LESO ==
  y : Inport
  u : Inport  Port=2
  Add : Sum  Inputs=+++
  Gain : Gain  Gain=3*wo_sep(ind)
  Gain1 : Gain  Gain=3*(wo_sep(ind))^2
  Gain2 : Gain  Gain=wo_sep(ind)^3
  Integrator : Integrator
  Integrator Limited : Integrator  LimitOutput=on  UpperSaturationLimit=25  LowerSaturationLimit=-25
  Integrator1 : Integrator
  Scope : Scope
  Sum : Sum  Inputs=|+-
  Sum1 : Sum  Inputs=|++
  err_leso_z : Scope
  Z1 : Outport
  Z2 : Outport  Port=2
  Z3 : Outport  Port=3
  wires:
  Gain/1 -> Sum1/1
  [Z1] -> Sum/2
  Gain1/1 -> Add/3
  Sum1/1 -> Integrator/1
  [Z2] -> Sum1/2
  Add/1 -> Integrator1/1
  Sum/1 -> err_leso_z/1, Gain/1, Gain1/1, Gain2/1
  Integrator/1 -> [Z1], Z1/1
  u/1 -> Add/2
  y/1 -> Sum/1
  [Z3] -> Add/1
  Gain2/1 -> Integrator Limited/1
  Integrator1/1 -> [Z2], Z2/1
  Integrator Limited/1 -> Z3/1, Scope/1, [Z3]

== system Control_v2/System/Controller/ADRC_Kalman/psi_loop/LESO ==
  y : Inport
  u : Inport  Port=2
  Add : Sum  Inputs=+++
  Gain : Gain  Gain=3*wo_sep(ind)
  Gain1 : Gain  Gain=3*(wo_sep(ind))^2
  Gain2 : Gain  Gain=wo_sep(ind)^3
  Integrator : Integrator
  Integrator Limited : Integrator  LimitOutput=on  UpperSaturationLimit=4  LowerSaturationLimit=-4
  Integrator1 : Integrator
  Integrator2 : Integrator
  Scope : Scope
  Sum : Sum  Inputs=|+-
  Sum1 : Sum  Inputs=|++
  err_leso_psi : Scope
  Z1 : Outport
  Z2 : Outport  Port=2
  Z3 : Outport  Port=3
  wires:
  Gain/1 -> Sum1/1
  [Z1] -> Sum/2
  Integrator2/1 -> Scope/1, [Z3], Z3/1
  Gain1/1 -> Add/3
  Sum1/1 -> Integrator/1
  [Z2] -> Sum1/2
  Add/1 -> Integrator1/1
  Sum/1 -> err_leso_psi/1, Gain/1, Gain1/1, Gain2/1
  Integrator/1 -> [Z1], Z1/1
  u/1 -> Add/2
  y/1 -> Sum/1
  [Z3] -> Add/1
  Gain2/1 -> Integrator2/1
  Integrator1/1 -> [Z2], Z2/1

== system Control_v2/System/Controller/ADRC_Kalman/theta_loop/LESO ==
  y : Inport
  u : Inport  Port=2
  Add : Sum  Inputs=+++
  Gain : Gain  Gain=3*wo_sep(ind)
  Gain1 : Gain  Gain=3*(wo_sep(ind))^2
  Gain2 : Gain  Gain=wo_sep(ind)^3
  Integrator : Integrator
  Integrator Limited : Integrator  LimitOutput=on  UpperSaturationLimit=4  LowerSaturationLimit=-4
  Integrator1 : Integrator
  Integrator2 : Integrator
  Sum : Sum  Inputs=|+-
  Sum1 : Sum  Inputs=|++
  z3_theta_scope : Scope
  Z1 : Outport
  Z2 : Outport  Port=2
  Z3 : Outport  Port=3
  wires:
  Integrator1/1 -> Z2/1, [Z2]
  Gain2/1 -> Integrator2/1
  [Z3] -> Add/1
  y/1 -> Sum/1
  u/1 -> Add/2
  Integrator/1 -> Z1/1, [Z1]
  Sum/1 -> Gain2/1, Gain1/1, Gain/1
  Add/1 -> Integrator1/1
  [Z2] -> Sum1/2
  Sum1/1 -> Integrator/1
  Gain1/1 -> Add/3
  Integrator2/1 -> z3_theta_scope/1, Z3/1, [Z3]
  [Z1] -> Sum/2
  Gain/1 -> Sum1/1

== system Control_v2/System/Controller/ADRC_SEP/Phi_loop/LESO ==
  y : Inport
  u : Inport  Port=2
  Add : Sum  Inputs=+++
  Gain : Gain  Gain=3*wo_sep(ind)
  Gain1 : Gain  Gain=3*(wo_sep(ind))^2
  Gain2 : Gain  Gain=wo_sep(ind)^3
  Integrator : Integrator
  Integrator Limited : Integrator  LimitOutput=on  UpperSaturationLimit=3  LowerSaturationLimit=-3
  Integrator1 : Integrator
  Integrator2 : Integrator
  Scope : Scope
  Sum : Sum  Inputs=|+-
  Sum1 : Sum  Inputs=|++
  Z1 : Outport
  Z2 : Outport  Port=2
  Z3 : Outport  Port=3
  wires:
  Integrator1/1 -> Z2/1, [Z2]
  [Z3] -> Add/1
  y/1 -> Sum/1
  u/1 -> Add/2
  Integrator/1 -> Z1/1, [Z1]
  Sum/1 -> Gain2/1, Gain1/1, Gain/1
  Add/1 -> Integrator1/1
  [Z2] -> Sum1/2
  Sum1/1 -> Integrator/1
  Gain1/1 -> Add/3
  Gain2/1 -> Integrator2/1
  [Z1] -> Sum/2
  Gain/1 -> Sum1/1
  Integrator2/1 -> Scope/1, Z3/1, [Z3]

== system Control_v2/System/Controller/ADRC_SEP/Z_loop/LESO ==
  y : Inport
  u : Inport  Port=2
  Add : Sum  Inputs=+++
  Gain : Gain  Gain=3*wo_sep(ind)
  Gain1 : Gain  Gain=3*(wo_sep(ind))^2
  Gain2 : Gain  Gain=wo_sep(ind)^3
  Integrator : Integrator
  Integrator Limited : Integrator  LimitOutput=on  UpperSaturationLimit=25  LowerSaturationLimit=-25
  Integrator1 : Integrator
  Scope : Scope
  Sum : Sum  Inputs=|+-
  Sum1 : Sum  Inputs=|++
  err_leso_z : Scope
  Z1 : Outport
  Z2 : Outport  Port=2
  Z3 : Outport  Port=3
  wires:
  Gain/1 -> Sum1/1
  [Z1] -> Sum/2
  Gain1/1 -> Add/3
  Sum1/1 -> Integrator/1
  [Z2] -> Sum1/2
  Add/1 -> Integrator1/1
  Sum/1 -> err_leso_z/1, Gain/1, Gain1/1, Gain2/1
  Integrator/1 -> [Z1], Z1/1
  u/1 -> Add/2
  y/1 -> Sum/1
  [Z3] -> Add/1
  Gain2/1 -> Integrator Limited/1
  Integrator1/1 -> [Z2], Z2/1
  Integrator Limited/1 -> Z3/1, Scope/1, [Z3]

== system Control_v2/System/Controller/ADRC_SEP/psi_loop/LESO ==
  y : Inport
  u : Inport  Port=2
  Add : Sum  Inputs=+++
  Gain : Gain  Gain=3*wo_sep(ind)
  Gain1 : Gain  Gain=3*(wo_sep(ind))^2
  Gain2 : Gain  Gain=wo_sep(ind)^3
  Integrator : Integrator
  Integrator Limited : Integrator  LimitOutput=on  UpperSaturationLimit=4  LowerSaturationLimit=-4
  Integrator1 : Integrator
  Integrator2 : Integrator
  Scope : Scope
  Sum : Sum  Inputs=|+-
  Sum1 : Sum  Inputs=|++
  err_leso_psi : Scope
  Z1 : Outport
  Z2 : Outport  Port=2
  Z3 : Outport  Port=3
  wires:
  Gain/1 -> Sum1/1
  [Z1] -> Sum/2
  Integrator2/1 -> Scope/1, [Z3], Z3/1
  Gain1/1 -> Add/3
  Sum1/1 -> Integrator/1
  [Z2] -> Sum1/2
  Add/1 -> Integrator1/1
  Sum/1 -> err_leso_psi/1, Gain/1, Gain1/1, Gain2/1
  Integrator/1 -> [Z1], Z1/1
  u/1 -> Add/2
  y/1 -> Sum/1
  [Z3] -> Add/1
  Gain2/1 -> Integrator2/1
  Integrator1/1 -> [Z2], Z2/1

== system Control_v2/System/Controller/ADRC_SEP/theta_loop/LESO ==
  y : Inport
  u : Inport  Port=2
  Add : Sum  Inputs=+++
  Gain : Gain  Gain=3*wo_sep(ind)
  Gain1 : Gain  Gain=3*(wo_sep(ind))^2
  Gain2 : Gain  Gain=wo_sep(ind)^3
  Integrator : Integrator
  Integrator Limited : Integrator  LimitOutput=on  UpperSaturationLimit=4  LowerSaturationLimit=-4
  Integrator1 : Integrator
  Integrator2 : Integrator
  Sum : Sum  Inputs=|+-
  Sum1 : Sum  Inputs=|++
  z3_theta_scope : Scope
  Z1 : Outport
  Z2 : Outport  Port=2
  Z3 : Outport  Port=3
  wires:
  Integrator1/1 -> Z2/1, [Z2]
  Gain2/1 -> Integrator2/1
  [Z3] -> Add/1
  y/1 -> Sum/1
  u/1 -> Add/2
  Integrator/1 -> Z1/1, [Z1]
  Sum/1 -> Gain2/1, Gain1/1, Gain/1
  Add/1 -> Integrator1/1
  [Z2] -> Sum1/2
  Sum1/1 -> Integrator/1
  Gain1/1 -> Add/3
  Integrator2/1 -> z3_theta_scope/1, Z3/1, [Z3]
  [Z1] -> Sum/2
  Gain/1 -> Sum1/1

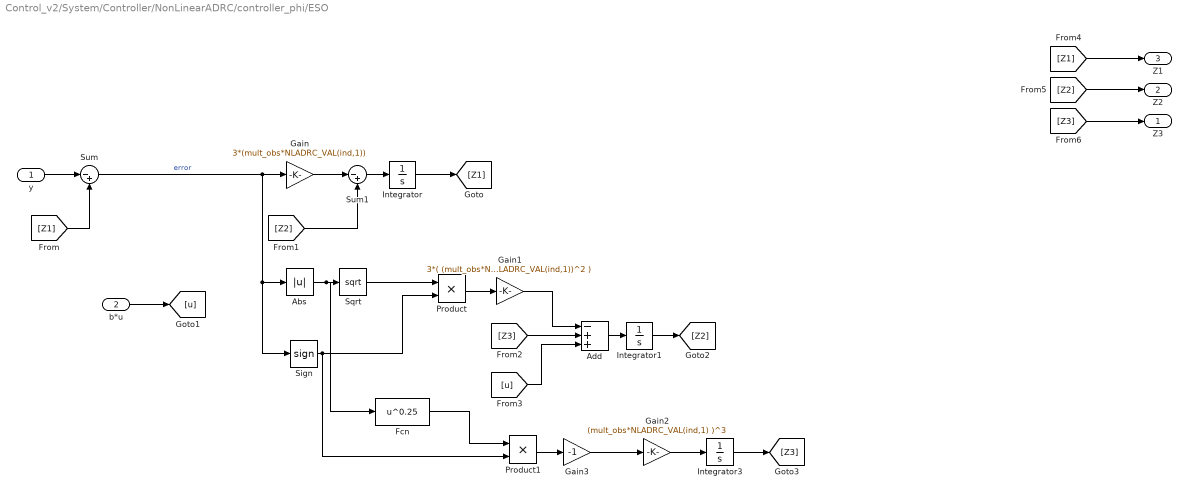
== system Control_v2/System/Controller/NonLinearADRC/controller_phi/ESO ==
  y : Inport
  b*u : Inport  Port=2
  Abs : Abs
  Add : Sum  Inputs=-++
  Fcn : Fcn  Expr=u^0.25
  Gain : Gain  Gain=3*(mult_obs*NLADRC_VAL(ind,1))
  Gain1 : Gain  Gain=3*( (mult_obs*NLADRC_VAL(ind,1))^2 )
  Gain2 : Gain  Gain=(mult_obs*NLADRC_VAL(ind,1) )^3
  Gain3 : Gain  Gain=-1
  Integrator : Integrator
  Integrator1 : Integrator
  Integrator3 : Integrator
  Product : Product
  Product1 : Product
  Sign : Signum
  Sqrt : Sqrt  SaturateOnIntegerOverflow=on
  Sum : Sum  Inputs=|-+
  Sum1 : Sum  Inputs=|-+
  Z3 : Outport
  Z2 : Outport  Port=2
  Z1 : Outport  Port=3
  wires:
  y/1 -> Sum/1
  [Z1] -> Sum/2
  Sum/1 -> Abs/1, Sign/1, Gain/1  "error"
  Gain/1 -> Sum1/1
  [Z2] -> Sum1/2
  Sum1/1 -> Integrator/1
  Integrator/1 -> [Z1]
  Abs/1 -> Fcn/1, Sqrt/1
  Sqrt/1 -> Product/1
  Sign/1 -> Product1/2, Product/2
  b*u/1 -> [u]
  Product/1 -> Gain1/1
  [Z3] -> Add/2
  [u] -> Add/3
  Add/1 -> Integrator1/1
  Integrator1/1 -> [Z2]
  Gain2/1 -> Integrator3/1
  Integrator3/1 -> [Z3]
  [Z1] -> Z1/1
  [Z2] -> Z2/1
  [Z3] -> Z3/1
  Gain1/1 -> Add/1
  Product1/1 -> Gain3/1
  Fcn/1 -> Product1/1
  Gain3/1 -> Gain2/1

== system Control_v2/System/Controller/NonLinearADRC/controller_phi/NLSEF ==
  e1 : Inport
  e2 : Inport  Port=2
  Scope : Scope  NumInputPorts=3
  Sum : Sum  Inputs=|++
  beta1_kp1 : Gain  Commented=on
  beta1_kp2 : Gain  Gain=NLADRC_VAL(ind,1)*NLADRC_VAL(ind,1)
  beta2_kd1 : Gain  Gain=2*epsi*NLADRC_VAL(ind,1)
  beta2_kd2 : Gain  Commented=on  Gain=0.01
  f_nl : Subsystem
  f_nl1 : Subsystem
  u : Outport
  wires:
  beta2_kd1/1 -> Sum/2  "kd"
  beta1_kp2/1 -> Sum/1  "kp"
  Sum/1 -> u/1
  e1/1 -> Scope/1, beta1_kp2/1
  e2/1 -> Scope/2, beta2_kd1/1

== system Control_v2/System/Controller/NonLinearADRC/controller_phi/TD ==
  v0 : Inport
  Abs : Abs
  Gain : Gain  Gain=1/(2*r(ind))
  Gain1 : Gain  Gain=-r(ind)
  Integrator : Integrator
  Integrator1 : Integrator
  Product : Product
  Sign : Signum
  Sum : Sum  Inputs=|++-
  Z1 : Outport
  Z2 : Outport  Port=2
  wires:
  Integrator/1 -> [Z1]
  [Z2] -> Integrator/1
  [Z1] -> Z1/1
  [Z2] -> Product/2, Abs/1
  Abs/1 -> Product/1
  Product/1 -> Gain/1
  [Z1] -> Sum/2
  Gain/1 -> Sum/1
  Integrator1/1 -> [Z2]
  [Z2] -> Z2/1
  v0/1 -> [v0]
  [v0] -> Sum/3
  Sum/1 -> Sign/1
  Sign/1 -> Gain1/1
  Gain1/1 -> Integrator1/1

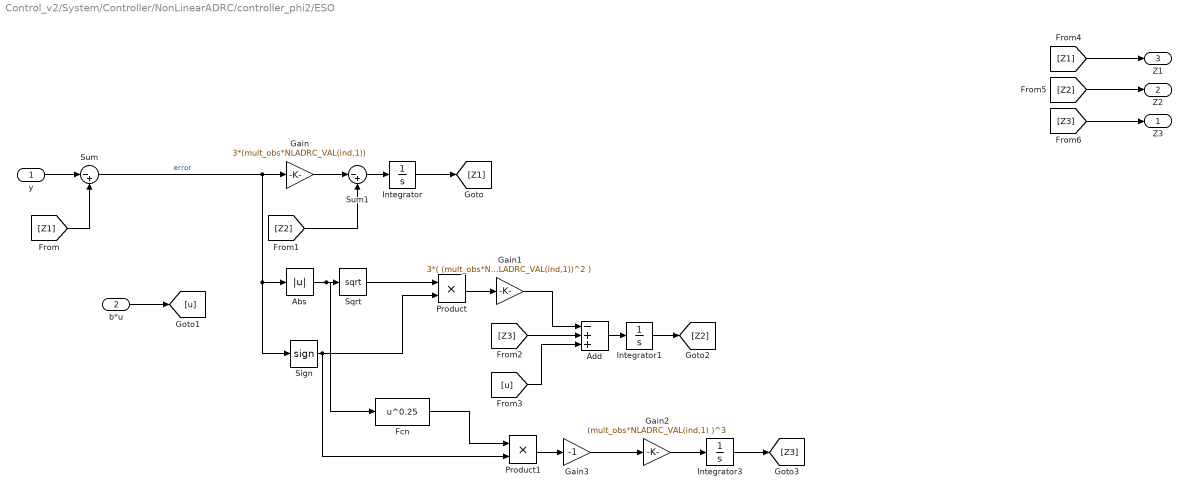
== system Control_v2/System/Controller/NonLinearADRC/controller_phi2/ESO ==
  y : Inport
  b*u : Inport  Port=2
  Abs : Abs
  Add : Sum  Inputs=-++
  Fcn : Fcn  Expr=u^0.25
  Gain : Gain  Gain=3*(mult_obs*NLADRC_VAL(ind,1))
  Gain1 : Gain  Gain=3*( (mult_obs*NLADRC_VAL(ind,1))^2 )
  Gain2 : Gain  Gain=(mult_obs*NLADRC_VAL(ind,1) )^3
  Gain3 : Gain  Gain=-1
  Integrator : Integrator
  Integrator1 : Integrator
  Integrator3 : Integrator
  Product : Product
  Product1 : Product
  Sign : Signum
  Sqrt : Sqrt  SaturateOnIntegerOverflow=on
  Sum : Sum  Inputs=|-+
  Sum1 : Sum  Inputs=|-+
  Z3 : Outport
  Z2 : Outport  Port=2
  Z1 : Outport  Port=3
  wires:
  y/1 -> Sum/1
  [Z1] -> Sum/2
  Sum/1 -> Abs/1, Sign/1, Gain/1  "error"
  Gain/1 -> Sum1/1
  [Z2] -> Sum1/2
  Sum1/1 -> Integrator/1
  Integrator/1 -> [Z1]
  Abs/1 -> Fcn/1, Sqrt/1
  Sqrt/1 -> Product/1
  Sign/1 -> Product1/2, Product/2
  b*u/1 -> [u]
  Product/1 -> Gain1/1
  [Z3] -> Add/2
  [u] -> Add/3
  Add/1 -> Integrator1/1
  Integrator1/1 -> [Z2]
  Gain2/1 -> Integrator3/1
  Integrator3/1 -> [Z3]
  [Z1] -> Z1/1
  [Z2] -> Z2/1
  [Z3] -> Z3/1
  Gain1/1 -> Add/1
  Product1/1 -> Gain3/1
  Fcn/1 -> Product1/1
  Gain3/1 -> Gain2/1

== system Control_v2/System/Controller/NonLinearADRC/controller_phi2/NLSEF ==
  e1 : Inport
  e2 : Inport  Port=2
  Scope : Scope  NumInputPorts=3
  Sum : Sum  Inputs=|++
  beta1_kp1 : Gain  Commented=on
  beta1_kp2 : Gain  Gain=NLADRC_VAL(ind,1)*NLADRC_VAL(ind,1)
  beta2_kd1 : Gain  Gain=2*epsi*NLADRC_VAL(ind,1)
  beta2_kd2 : Gain  Commented=on  Gain=0.01
  f_nl : Subsystem
  f_nl1 : Subsystem
  u : Outport
  wires:
  Sum/1 -> u/1
  beta1_kp2/1 -> Sum/1  "kp"
  beta2_kd1/1 -> Sum/2  "kd"
  e1/1 -> beta1_kp2/1
  e2/1 -> beta2_kd1/1

== system Control_v2/System/Controller/NonLinearADRC/controller_phi2/TD ==
  v0 : Inport
  Abs : Abs
  Gain : Gain  Gain=1/(2*r(ind))
  Gain1 : Gain  Gain=-r(ind)
  Integrator : Integrator
  Integrator1 : Integrator
  Product : Product
  Sign : Signum
  Sum : Sum  Inputs=|++-
  Z1 : Outport
  Z2 : Outport  Port=2
  wires:
  Integrator/1 -> [Z1]
  [Z2] -> Integrator/1
  [Z1] -> Z1/1
  [Z2] -> Product/2, Abs/1
  Abs/1 -> Product/1
  Product/1 -> Gain/1
  [Z1] -> Sum/2
  Gain/1 -> Sum/1
  Integrator1/1 -> [Z2]
  [Z2] -> Z2/1
  v0/1 -> [v0]
  [v0] -> Sum/3
  Sum/1 -> Sign/1
  Sign/1 -> Gain1/1
  Gain1/1 -> Integrator1/1

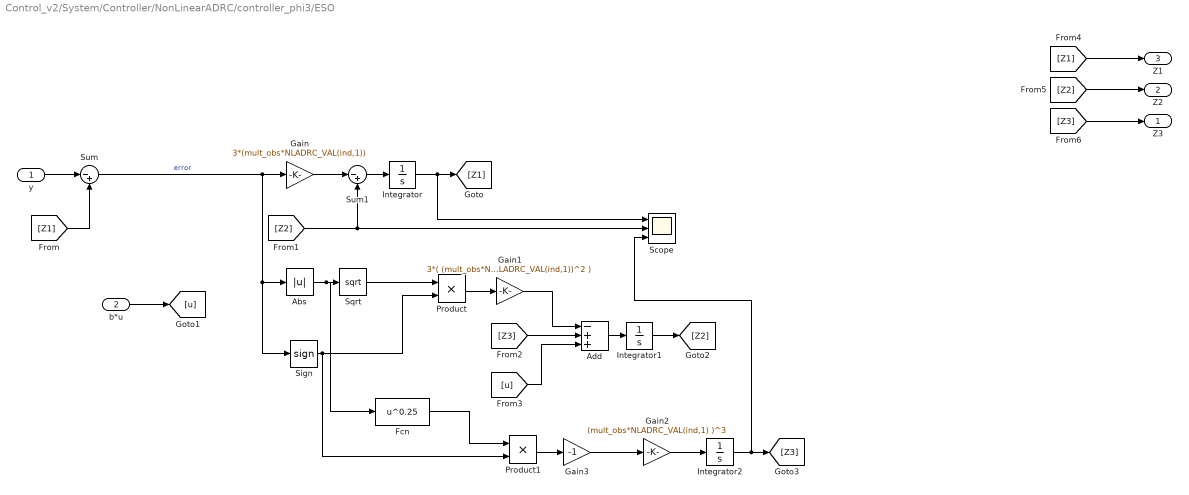
== system Control_v2/System/Controller/NonLinearADRC/controller_phi3/ESO ==
  y : Inport
  b*u : Inport  Port=2
  Abs : Abs
  Add : Sum  Inputs=-++
  Fcn : Fcn  Expr=u^0.25
  Gain : Gain  Gain=3*(mult_obs*NLADRC_VAL(ind,1))
  Gain1 : Gain  Gain=3*( (mult_obs*NLADRC_VAL(ind,1))^2 )
  Gain2 : Gain  Gain=(mult_obs*NLADRC_VAL(ind,1) )^3
  Gain3 : Gain  Gain=-1
  Integrator : Integrator
  Integrator1 : Integrator
  Integrator2 : Integrator
  Product : Product
  Product1 : Product
  Scope : Scope  NumInputPorts=3
  Sign : Signum
  Sqrt : Sqrt  SaturateOnIntegerOverflow=on
  Sum : Sum  Inputs=|-+
  Sum1 : Sum  Inputs=|-+
  Z3 : Outport
  Z2 : Outport  Port=2
  Z1 : Outport  Port=3
  wires:
  Gain3/1 -> Gain2/1
  Fcn/1 -> Product1/1
  Product1/1 -> Gain3/1
  Gain1/1 -> Add/1
  [Z3] -> Z3/1
  [Z2] -> Z2/1
  [Z1] -> Z1/1
  Gain2/1 -> Integrator2/1
  Integrator1/1 -> [Z2]
  Add/1 -> Integrator1/1
  [u] -> Add/3
  [Z3] -> Add/2
  Product/1 -> Gain1/1
  b*u/1 -> [u]
  Sign/1 -> Product/2, Product1/2
  Sqrt/1 -> Product/1
  Abs/1 -> Sqrt/1, Fcn/1
  Sum1/1 -> Integrator/1
  [Z2] -> Sum1/2, Scope/2
  Gain/1 -> Sum1/1
  Sum/1 -> Gain/1, Sign/1, Abs/1  "error"
  [Z1] -> Sum/2
  y/1 -> Sum/1
  Integrator/1 -> Scope/1, [Z1]
  Integrator2/1 -> Scope/3, [Z3]

== system Control_v2/System/Controller/NonLinearADRC/controller_phi3/NLSEF ==
  e1 : Inport
  e2 : Inport  Port=2
  Scope : Scope  NumInputPorts=3
  Sum : Sum  Inputs=|++
  beta1_kp1 : Gain  Commented=on
  beta1_kp2 : Gain  Gain=NLADRC_VAL(ind,1)*NLADRC_VAL(ind,1)
  beta2_kd1 : Gain  Gain=2*epsi*NLADRC_VAL(ind,1)
  beta2_kd2 : Gain  Commented=on  Gain=0.01
  f_nl : Subsystem
  f_nl1 : Subsystem
  u : Outport
  wires:
  Sum/1 -> u/1
  beta1_kp2/1 -> Sum/1  "kp"
  beta2_kd1/1 -> Sum/2  "kd"
  e1/1 -> Scope/1, beta1_kp2/1
  e2/1 -> Scope/2, beta2_kd1/1

== system Control_v2/System/Controller/NonLinearADRC/controller_phi3/TD ==
  v0 : Inport
  Abs : Abs
  Gain : Gain  Gain=1/(2*r(ind))
  Gain1 : Gain  Gain=-r(ind)
  Integrator : Integrator
  Integrator1 : Integrator
  Product : Product
  Sign : Signum
  Sum : Sum  Inputs=|++-
  Z1 : Outport
  Z2 : Outport  Port=2
  wires:
  Gain1/1 -> Integrator1/1
  Sign/1 -> Gain1/1
  Sum/1 -> Sign/1
  [v0] -> Sum/3
  v0/1 -> [v0]
  [Z2] -> Z2/1
  Integrator1/1 -> [Z2]
  Gain/1 -> Sum/1
  [Z1] -> Sum/2
  Product/1 -> Gain/1
  Abs/1 -> Product/1
  [Z2] -> Abs/1, Product/2
  [Z1] -> Z1/1
  [Z2] -> Integrator/1
  Integrator/1 -> [Z1]

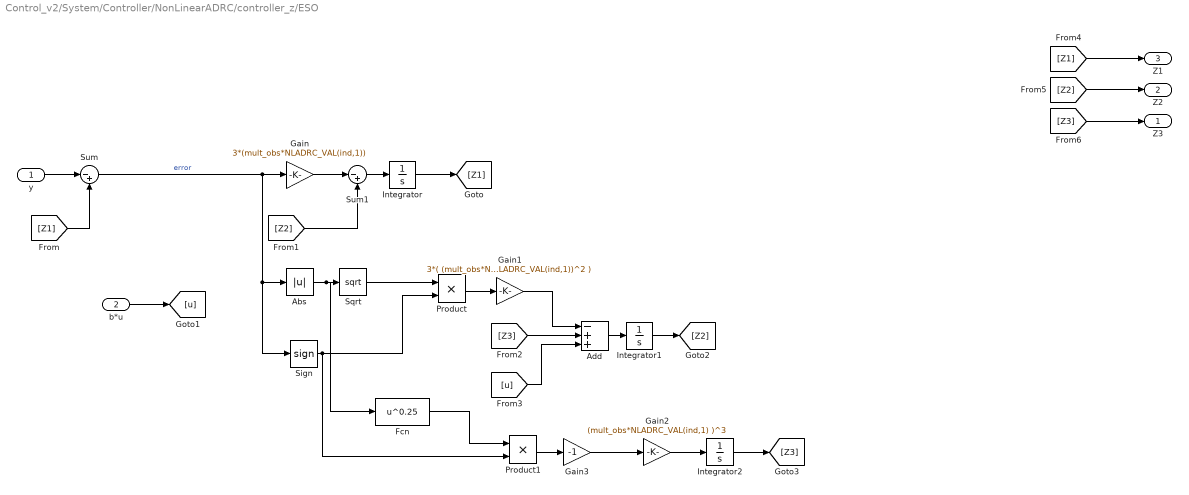
== system Control_v2/System/Controller/NonLinearADRC/controller_z/ESO ==
  y : Inport
  b*u : Inport  Port=2
  Abs : Abs
  Add : Sum  Inputs=-++
  Fcn : Fcn  Expr=u^0.25
  Gain : Gain  Gain=3*(mult_obs*NLADRC_VAL(ind,1))
  Gain1 : Gain  Gain=3*( (mult_obs*NLADRC_VAL(ind,1))^2 )
  Gain2 : Gain  Gain=(mult_obs*NLADRC_VAL(ind,1) )^3
  Gain3 : Gain  Gain=-1
  Integrator : Integrator
  Integrator1 : Integrator
  Integrator2 : Integrator
  Product : Product
  Product1 : Product
  Sign : Signum
  Sqrt : Sqrt  SaturateOnIntegerOverflow=on
  Sum : Sum  Inputs=|-+
  Sum1 : Sum  Inputs=|-+
  Z3 : Outport
  Z2 : Outport  Port=2
  Z1 : Outport  Port=3
  wires:
  Gain3/1 -> Gain2/1
  Fcn/1 -> Product1/1
  Product1/1 -> Gain3/1
  Gain1/1 -> Add/1
  [Z3] -> Z3/1
  [Z2] -> Z2/1
  [Z1] -> Z1/1
  Integrator2/1 -> [Z3]
  Gain2/1 -> Integrator2/1
  Integrator1/1 -> [Z2]
  Add/1 -> Integrator1/1
  [u] -> Add/3
  [Z3] -> Add/2
  Product/1 -> Gain1/1
  b*u/1 -> [u]
  Sign/1 -> Product/2, Product1/2
  Sqrt/1 -> Product/1
  Abs/1 -> Sqrt/1, Fcn/1
  Integrator/1 -> [Z1]
  Sum1/1 -> Integrator/1
  [Z2] -> Sum1/2
  Gain/1 -> Sum1/1
  Sum/1 -> Gain/1, Sign/1, Abs/1  "error"
  [Z1] -> Sum/2
  y/1 -> Sum/1

== system Control_v2/System/Controller/NonLinearADRC/controller_z/NLSEF ==
  e1 : Inport
  e2 : Inport  Port=2
  Scope : Scope  NumInputPorts=3
  Sum : Sum  Inputs=|++
  beta1_kp1 : Gain  Commented=on
  beta1_kp2 : Gain  Gain=NLADRC_VAL(ind,1)*NLADRC_VAL(ind,1)
  beta2_kd1 : Gain  Gain=2*epsi*NLADRC_VAL(ind,1)
  beta2_kd2 : Gain  Commented=on  Gain=0.01
  f_nl : Subsystem
  f_nl1 : Subsystem
  u : Outport
  wires:
  beta2_kd1/1 -> Sum/2  "kd"
  beta1_kp2/1 -> Sum/1  "kp"
  Sum/1 -> u/1
  e1/1 -> beta1_kp2/1, Scope/1
  e2/1 -> Scope/2, beta2_kd1/1

== system Control_v2/System/Controller/NonLinearADRC/controller_z/TD ==
  v0 : Inport
  Abs : Abs
  Gain : Gain  Gain=1/(2*r(ind))
  Gain1 : Gain  Gain=-r(ind)
  Integrator : Integrator
  Integrator1 : Integrator
  Product : Product
  sat : MATLAB Function  TreatAsAtomicUnit=on
  Z1 : Outport
  Z2 : Outport  Port=2
  wires:
  Gain1/1 -> Integrator1/1
  sat/1(y) -> Gain1/1
  v0/1 -> [v0]
  [Z2] -> Z2/1
  Integrator1/1 -> [Z2]
  Product/1 -> Gain/1
  Abs/1 -> Product/1
  [Z2] -> Abs/1, Product/2
  [Z1] -> Z1/1
  [Z2] -> Integrator/1
  Integrator/1 -> [Z1]
  [Z1] -> sat/1(x1)
  [v0] -> sat/2(v0)
  Gain/1 -> sat/3(x2)

== system Control_v2/System/Controller/NonLinearADRC/controller_phi/NLSEF/f_nl ==
  e : Inport
  Constant2 : Constant
  Divide : Product  Inputs=*/
  Power : Math  Operator=pow  SignedPower=off  SaturateOnIntegerOverflow=on
  Power1 : Math  Operator=pow  SignedPower=off  SaturateOnIntegerOverflow=on
  Product : Product
  Sign1 : Signum
  Subtract : Sum  Inputs=+-
  Switch : Switch  Criteria=u2 > Threshold  Threshold=NLADRC_VAL(ind,2)
  eta : Constant  Value=NLADRC_VAL(ind,2)
  gamma : Constant  Value=NLADRC_VAL(ind,3)
  fnl : Outport
  wires:
  [err] -> Divide/1
  Sign1/1 -> [sign_err]
  [abs_err] -> Switch/2
  Product/1 -> Switch/1
  e/1 -> Sign1/1, [abs_err], [err]
  Constant2/1 -> Subtract/2
  Power/1 -> Product/1
  [sign_err] -> Product/2
  eta/1 -> Power1/1
  Subtract/1 -> Power1/2
  Power1/1 -> Divide/2
  Divide/1 -> Switch/3
  [abs_err] -> Power/1
  gamma/1 -> Power/2, Subtract/1
  Switch/1 -> fnl/1

== system Control_v2/System/Controller/NonLinearADRC/controller_phi/NLSEF/f_nl1 ==
  e : Inport
  Constant2 : Constant
  Divide : Product  Inputs=*/
  Power : Math  Operator=pow  SignedPower=off  SaturateOnIntegerOverflow=on
  Power1 : Math  Operator=pow  SignedPower=off  SaturateOnIntegerOverflow=on
  Product : Product
  Sign1 : Signum
  Subtract : Sum  Inputs=+-
  Switch : Switch  Criteria=u2 > Threshold  Threshold=NLADRC_VAL(ind,2)
  eta : Constant  Value=NLADRC_VAL(ind,2)
  gamma : Constant  Value=NLADRC_VAL(ind,3)
  fnl : Outport
  wires:
  Switch/1 -> fnl/1
  gamma/1 -> Subtract/1, Power/2
  [abs_err] -> Power/1
  Divide/1 -> Switch/3
  Power1/1 -> Divide/2
  Subtract/1 -> Power1/2
  eta/1 -> Power1/1
  [sign_err] -> Product/2
  Power/1 -> Product/1
  Constant2/1 -> Subtract/2
  e/1 -> [err], [abs_err], Sign1/1
  Product/1 -> Switch/1
  [abs_err] -> Switch/2
  Sign1/1 -> [sign_err]
  [err] -> Divide/1

== system Control_v2/System/Controller/NonLinearADRC/controller_phi2/NLSEF/f_nl ==
  e : Inport
  Constant2 : Constant
  Divide : Product  Inputs=*/
  Power : Math  Operator=pow  SignedPower=off  SaturateOnIntegerOverflow=on
  Power1 : Math  Operator=pow  SignedPower=off  SaturateOnIntegerOverflow=on
  Product : Product
  Sign1 : Signum
  Subtract : Sum  Inputs=+-
  Switch : Switch  Criteria=u2 > Threshold  Threshold=NLADRC_VAL(ind,2)
  eta : Constant  Value=NLADRC_VAL(ind,2)
  gamma : Constant  Value=NLADRC_VAL(ind,3)
  fnl : Outport
  wires:
  [err] -> Divide/1
  Sign1/1 -> [sign_err]
  [abs_err] -> Switch/2
  Product/1 -> Switch/1
  e/1 -> Sign1/1, [abs_err], [err]
  Constant2/1 -> Subtract/2
  Power/1 -> Product/1
  [sign_err] -> Product/2
  eta/1 -> Power1/1
  Subtract/1 -> Power1/2
  Power1/1 -> Divide/2
  Divide/1 -> Switch/3
  [abs_err] -> Power/1
  gamma/1 -> Power/2, Subtract/1
  Switch/1 -> fnl/1
